simulink library "TriphaseHardwaremodule"  (R2019b)
settings: Solver=ode45  StartTime=0.0  StopTime=10.0  RelTol=1e-3
values from neighbouring files (symbols this model uses):
  ControlSampleTime = 1/8000    (= 0.000125)    [initTPHardware.m]
  HWSampleTime = ControlSampleTime / Oversample    [Sim_TP3_VSM_init.m]    (also in initTPHardware.m = 3.125e-05)
  L1 = 0    [initVirtualCircuit.m]
undefined symbols (not defined in the file or in its folder): C1, C2, C_cap, C_CM, C_damp, C_DC, DT, gcbh, Iac_bit, Iac_max, L2, L_CM, LCL, PWM_f, R_C1, R_C2, R_cap, R_damp, R_L1, R_L2, sps_rtmsupport, Vac_bit, Vac_max, Vdc_bit, Vdc_max
libraries: $bdroot x58, powerlib x46, triphase_hpc x7, powerlib_meascontrol x5, simulink x2
(part 1 of 3)
settings Model: Creator=fwelck  LastModifiedBy=e2n016
settings DataIOCC: LimitDataPoints=on  SaveFormat=Array  ReturnWorkspaceOutputs=off
settings OptimizationCC: BlockReduction=off  BooleanDataType=off  LifeSpan=inf
settings DebuggingCC: SaveWithParameterizedLinksMsg=none  UnderspecifiedInitializationDetection=Classic  MergeDetectMultiDrivingBlocksExec=none  SignalResolutionControl=TryResolveAllWithWarning  AllowSymbolicDim=off  SFUnexpectedBacktrackingDiag=warning  SFNoUnconditionalDefaultTransitionDiag=warning  SFExecutionAtInitializationDiag=none  ArithmeticOperatorsInVariantConditions=warning
settings HardwareCC: ProdBitPerPointer=32  ProdBitPerSizeT=32  ProdBitPerPtrDiffT=32  ProdLargestAtomicFloat=None  ProdIntDivRoundTo=Undefined  ProdEndianess=Unspecified  ProdWordSize=32  ProdHWDeviceType=32-bit Generic  TargetUnknown=on
settings ModelReferenceCC: PropagateSignalLabelsOutOfModel=off
settings SFSimCC: SimUseLocalCustomCode=off  CustomCodeUndefinedFunction=UseInterfaceOnly
settings RTWCC: RTWUseLocalCustomCode=off
settings CodeAppCC: StateflowObjectComments=on
settings GRTTargetCC: TargetLangStandard=C89/C90 (ANSI)  GeneratePreprocessorConditionals=Disable all
settings ConfigComp: CovMetricSettings=dw  CovHtmlReporting=on  CovSaveCumulativeToWorkspaceVar=on  CovSaveSingleToWorkspaceVar=on  CovExternalEMLEnable=off  CovSFcnEnable=off

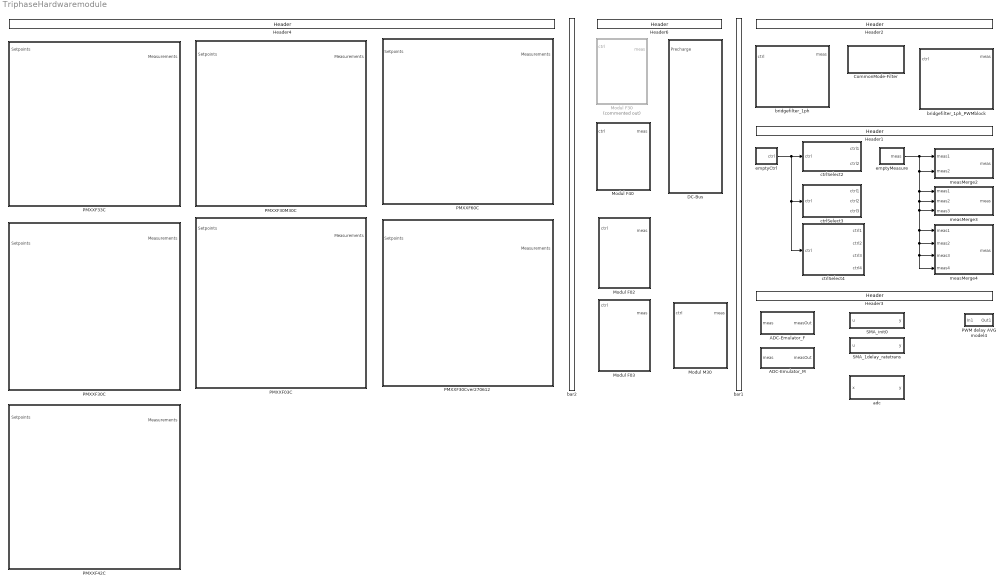
== system TriphaseHardwaremodule ==
  ADC-Emulator_F : Subsystem  mask{ADC_Emulation=off, ControlSampleTime=ControlSampleTime, HWSampleTime=HWSampleTime, Vac_max=Vac_max, Vac_bit=Vac_bit, Iac_max=Iac_max, Iac_bit=Iac_bit, Vdc_max=Vdc_max, Vdc_bit=Vdc_bit}
      mask prompts: Vac_max "AC Voltage Range"; Vac_bit "ADC resolution [bit]"; Iac_max "AC Current Range"; Iac_bit "ADC resolution [bit]"; Vdc_max "DC Voltage Range"; Vdc_bit "ADC resolution [bit]"
      mask init:
      | ParamValue=get_param(gcb,'ADC_Emulation');
      | set_param([gcb '/adc_i_inverter'],'ADC_Emulation',ParamValue);
      | set_param([gcb '/adc_i_out'],'ADC_Emulation',ParamValue);
      | set_param([gcb '/adc_u_cap'],'ADC_Emulation',ParamValue);
      | set_param([gcb '/adc_u_dc'],'ADC_Emulation',ParamValue);
      | set_param([gcb '/adc_u_out'],'ADC_Emulation',ParamValue);
      mask TypeOptions ADC_Emulation: off | on
      mask DialogControl GrpADC Prompt: ADC-Emulation
      mask DialogControl ADC_Text Prompt: ADC-emulation emulates the quantization resulting from AD-conversion. Moving Average is always applied over one ControlSampleTime
  ADC-Emulator_M : Subsystem  mask{ADC_Emulation=off, ControlSampleTime=ControlSampleTime, HWSampleTime=HWSampleTime, Vac_max=Vac_max, Vac_bit=Vac_bit, Iac_max=Iac_max, Iac_bit=Iac_bit, Vdc_max=Vdc_max, Vdc_bit=Vdc_bit}
      mask prompts: Vac_max "AC Voltage Range"; Vac_bit "ADC resolution [bit]"; Iac_max "AC Current Range"; Iac_bit "ADC resolution [bit]"; Vdc_max "DC Voltage Range"; Vdc_bit "ADC resolution [bit]"
      mask init:
      | ParamValue=get_param(gcb,'ADC_Emulation');
      | set_param([gcb '/adc_i_inverter'],'ADC_Emulation',ParamValue);
      | set_param([gcb '/adc_u_dc'],'ADC_Emulation',ParamValue);
      mask TypeOptions ADC_Emulation: off | on
      mask DialogControl GrpADC Prompt: ADC-Emulation
      mask DialogControl ADC_Text Prompt: ADC-emulation emulates the quantization resulting from AD-conversion. Moving Average is always applied over one ControlSampleTime
  CommonMode-Filter : Subsystem  mask{L_CM=L_CM, C_CM=C_CM, R_damp=R_damp, C_damp=C_damp}
      mask prompts: L_CM "Inductance [H]"; C_CM "Capacitance [F]"; R_damp "Damping resistance [Ohm]"; C_damp "Damping capacitance [F]"
      mask DialogControl GrpCM Prompt: Common-Mode
  DC-Bus : Subsystem  mask{C_cap=C_cap, R_cap=R_cap}
      mask prompts: C_cap "Capacitance [F]"; R_cap "Parallel Resistance [Ohm]"
      mask DialogControl GrpDC Prompt: DC-Bus
  Header1 : triphase_hpc/Utilities/Header  strCap=Signal Split and Merge  strColor=Dark Gray  strPen=white
  Header2 : triphase_hpc/Utilities/Header  strCap=Basic Inverter Modules  strColor=Dark Gray  strPen=white
  Header3 : triphase_hpc/Utilities/Header  strCap=ADC Modules  strColor=Dark Gray  strPen=white
  Header4 : triphase_hpc/Utilities/Header  strCap=Triphase Hardware  strColor=Dark Gray  strPen=white
  Header6 : triphase_hpc/Utilities/Header  strCap=Basic Triphase Modules  strColor=Dark Gray  strPen=white
  Modul F02 : Subsystem  mask{Leistungsklasse=Custom, LCFilterChoice=LC, L1=L1, R_L1=R_L1, C1=C1, R_C1=R_C1, L2=L2, R_L2=R_L2, C2=C2, R_C2=R_C2, PWM_f=PWM_f, DT=DT, ADC_Emulation=off, ControlSampleTime=ControlSampleTime, HWSampleTime=HWSampleTime, Vac_max=Vac_max, Vac_bit=Vac_bit, Iac_max=Iac_max, Iac_bit=Iac_bit, Vdc_max=Vdc_max, Vdc_bit=Vdc_bit}
      mask prompts: LCFilterChoice "AC-Filter"; L1 "Inductance L1 [H]"; R_L1 "Series resistance of L1 [Ohm]"; C1 "Capacitance C1 [F]"; R_C1 "Series resistance of C1 [Ohm]"; L2 "Inductance L2 [H]"; R_L2 "Series resistance of L2 [Ohm]"; C2 "Capacitance C2 [F]"; R_C2 "Series resistance of C2 [Ohm]"; PWM_f "PWM Frequency"; DT "On Delay"; Vac_max "AC Voltage Range"; Vac_bit "ADC resolution [bit]"; Iac_max "AC Current Range"; Iac_bit "ADC resolution [bit]"; Vdc_max "DC Voltage Range"; Vdc_bit "ADC resolution [bit]"
      mask init:
      | ParamValue=get_param(gcb,'ADC_Emulation');
      | set_param([gcb '/ADC-Emulator_F'],'ADC_Emulation',ParamValue);
      | 
      | ParamValue=get_param(gcb,'LCFilterChoice');
      | set_param([gcb '/bridgefilter_dca'],'LCFilterChoice',ParamValue);
      | set_param([gcb '/bridgefilter_dcb'],'LCFilterChoice',ParamValue);
      mask TypeOptions Leistungsklasse: 5kW | 15kW | 90kW | Custom
      mask Callback Leistungsklasse: loadTriphaseHardwareParameter
      mask TypeOptions LCFilterChoice: LC | LCL | LCC | LCLC
      mask TypeOptions ADC_Emulation: off | on
      mask DialogControl GrpLoad Prompt: Triphase
      mask DialogControl LC Prompt: LC(L)(C)
      mask DialogControl GrpLC Prompt: LC(L)(C)-Filter
      mask DialogControl SW Prompt: Swichted
      mask DialogControl GrpSW Prompt: Switched
      mask DialogControl ADC Prompt: ADC
      mask DialogControl GrpADC Prompt: ADC-Emulation
      mask DialogControl ADC_Text Prompt: ADC-emulation emulates the quantization resulting from AD-conversion. Moving Average is always applied over one ControlSampleTime
  Modul F03 : Subsystem  mask{Leistungsklasse=Custom, LCFilterChoice=LC, L1=L1, R_L1=R_L1, C1=C1, R_C1=R_C1, L2=L2, R_L2=R_L2, C2=C2, R_C2=R_C2, PWM_f=PWM_f, DT=DT, ADC_Emulation=off, ControlSampleTime=ControlSampleTime, HWSampleTime=HWSampleTime, Vac_max=Vac_max, Vac_bit=Vac_bit, Iac_max=Iac_max, Iac_bit=Iac_bit, Vdc_max=Vdc_max, Vdc_bit=Vdc_bit}
      mask prompts: LCFilterChoice "AC-Filter"; L1 "Inductance L1 [H]"; R_L1 "Series resistance of L1 [Ohm]"; C1 "Capacitance C1 [F]"; R_C1 "Series resistance of C1 [Ohm]"; L2 "Inductance L2 [H]"; R_L2 "Series resistance of L2 [Ohm]"; C2 "Capacitance C2 [F]"; R_C2 "Series resistance of C2 [Ohm]"; PWM_f "PWM Frequency"; DT "On Delay"; Vac_max "AC Voltage Range"; Vac_bit "ADC resolution [bit]"; Iac_max "AC Current Range"; Iac_bit "ADC resolution [bit]"; Vdc_max "DC Voltage Range"; Vdc_bit "ADC resolution [bit]"
      mask init:
      | ParamValue=get_param(gcb,'ADC_Emulation');
      | set_param([gcb '/ADC-Emulator_F'],'ADC_Emulation',ParamValue);
      | 
      | ParamValue=get_param(gcb,'LCFilterChoice');
      | set_param([gcb '/bridgefilter_dca'],'LCFilterChoice',ParamValue);
      | set_param([gcb '/bridgefilter_dcb'],'LCFilterChoice',ParamValue);
      | set_param([gcb '/bridgefilter_dcb1'],'LCFilterChoice',ParamValue);
      mask TypeOptions Leistungsklasse: 5kW | 15kW | 90kW | Custom
      mask Callback Leistungsklasse: loadTriphaseHardwareParameter
      mask TypeOptions LCFilterChoice: LC | LCL | LCC | LCLC
      mask TypeOptions ADC_Emulation: off | on
      mask DialogControl GrpLoad Prompt: Triphase
      mask DialogControl LC Prompt: LC(L)(C)
      mask DialogControl GrpLC Prompt: LC(L)(C)-Filter
      mask DialogControl SW Prompt: Swichted
      mask DialogControl GrpSW Prompt: Switched
      mask DialogControl ADC Prompt: ADC
      mask DialogControl GrpADC Prompt: ADC-Emulation
      mask DialogControl ADC_Text Prompt: ADC-emulation emulates the quantization resulting from AD-conversion. Moving Average is always applied over one ControlSampleTime
  Modul F30 : Subsystem  Commented=on  mask{Leistungsklasse=Custom, LCFilterChoice=LCLC, L1=L1, R_L1=R_L1, C1=C1, R_C1=R_C1, L2=L2, R_L2=R_L2, C2=C2, R_C2=R_C2, PWM_f=PWM_f, DT=DT, ADC_Emulation=off, ControlSampleTime=ControlSampleTime, HWSampleTime=HWSampleTime, Vac_max=Vac_max, Vac_bit=Vac_bit, Iac_max=Iac_max, Iac_bit=Iac_bit, Vdc_max=Vdc_max, Vdc_bit=Vdc_bit}
      mask prompts: LCFilterChoice "AC-Filter"; L1 "Inductance L1 [H]"; R_L1 "Series resistance of L1 [Ohm]"; C1 "Capacitance C1 [F]"; R_C1 "Series resistance of C1 [Ohm]"; L2 "Inductance L2 [H]"; R_L2 "Series resistance of L2 [Ohm]"; C2 "Capacitance C2 [F]"; R_C2 "Series resistance of C2 [Ohm]"; PWM_f "PWM Frequency"; DT "On Delay"; Vac_max "AC Voltage Range"; Vac_bit "ADC resolution [bit]"; Iac_max "AC Current Range"; Iac_bit "ADC resolution [bit]"; Vdc_max "DC Voltage Range"; Vdc_bit "ADC resolution [bit]"
      mask init:
      | ParamValue=get_param(gcb,'ADC_Emulation');
      | set_param([gcb '/ADC-Emulator_F'],'ADC_Emulation',ParamValue);
      | 
      | ParamValue=get_param(gcb,'LCFilterChoice');
      | set_param([gcb '/bridgefilter_aca'],'LCFilterChoice',ParamValue);
      | set_param([gcb '/bridgefilter_acb'],'LCFilterChoice',ParamValue);
      | set_param([gcb '/bridgefilter_acc'],'LCFilterChoice',ParamValue);
      mask TypeOptions Leistungsklasse: 5kW | 15kW | 90kW | Custom
      mask Callback Leistungsklasse: loadTriphaseHardwareParameter
      mask TypeOptions LCFilterChoice: LC | LCL | LCC | LCLC
      mask TypeOptions ADC_Emulation: off | on
      mask DialogControl GrpLoad Prompt: Triphase
      mask DialogControl LC Prompt: LC(L)(C)
      mask DialogControl GrpLC Prompt: LC(L)(C)-Filter
      mask DialogControl SW Prompt: Swichted
      mask DialogControl GrpSW Prompt: Switched
      mask DialogControl ADC Prompt: ADC
      mask DialogControl GrpADC Prompt: ADC-Emulation
      mask DialogControl ADC_Text Prompt: ADC-emulation emulates the quantization resulting from AD-conversion. Moving Average is always applied over one ControlSampleTime
  Modul F40 : Subsystem  mask{Leistungsklasse=Custom, LCFilterChoice=LC, L1=L1, R_L1=R_L1, C1=C1, R_C1=R_C1, L2=L2, R_L2=R_L2, C2=C2, R_C2=R_C2, PWM_f=PWM_f, DT=DT, ADC_Emulation=off, ControlSampleTime=ControlSampleTime, HWSampleTime=HWSampleTime, Vac_max=Vac_max, Vac_bit=Vac_bit, Iac_max=Iac_max, Iac_bit=Iac_bit, Vdc_max=Vdc_max, Vdc_bit=Vdc_bit}
      mask prompts: LCFilterChoice "AC-Filter"; L1 "Inductance L1 [H]"; R_L1 "Series resistance of L1 [Ohm]"; C1 "Capacitance C1 [F]"; R_C1 "Series resistance of C1 [Ohm]"; L2 "Inductance L2 [H]"; R_L2 "Series resistance of L2 [Ohm]"; C2 "Capacitance C2 [F]"; R_C2 "Series resistance of C2 [Ohm]"; PWM_f "PWM Frequency"; DT "On Delay"; Vac_max "AC Voltage Range"; Vac_bit "ADC resolution [bit]"; Iac_max "AC Current Range"; Iac_bit "ADC resolution [bit]"; Vdc_max "DC Voltage Range"; Vdc_bit "ADC resolution [bit]"
      mask init:
      | ParamValue=get_param(gcb,'ADC_Emulation');
      | set_param([gcb '/ADC-Emulator_F'],'ADC_Emulation',ParamValue);
      | 
      | ParamValue=get_param(gcb,'LCFilterChoice');
      | set_param([gcb '/bridgefilter_aca'],'LCFilterChoice',ParamValue);
      | set_param([gcb '/bridgefilter_acb'],'LCFilterChoice',ParamValue);
      | set_param([gcb '/bridgefilter_acc'],'LCFilterChoice',ParamValue);
      | set_param([gcb '/bridgefilter_acd'],'LCFilterChoice',ParamValue);
      mask TypeOptions Leistungsklasse: 5kW | 15kW | 90kW | Custom
      mask Callback Leistungsklasse: loadTriphaseHardwareParameter
      mask TypeOptions LCFilterChoice: LC | LCL | LCC | LCLC
      mask TypeOptions ADC_Emulation: off | on
      mask DialogControl GrpLoad Prompt: Triphase
      mask DialogControl LC Prompt: LC(L)(C)
      mask DialogControl GrpLC Prompt: LC(L)(C)-Filter
      mask DialogControl SW Prompt: Swichted
      mask DialogControl GrpSW Prompt: Switched
      mask DialogControl ADC Prompt: ADC
      mask DialogControl GrpADC Prompt: ADC-Emulation
      mask DialogControl ADC_Text Prompt: ADC-emulation emulates the quantization resulting from AD-conversion. Moving Average is always applied over one ControlSampleTime
  Modul M30 : Subsystem  mask{PWM_f=PWM_f, DT=DT}
      mask prompts: PWM_f "PWM Frequency"; DT "On Delay"
      mask DialogControl GrpSW Prompt: Switched
  PMXXF03C : Subsystem  VariantControl=PMXXF03C  mask{Leistungsklasse=Custom, LCFilterChoice=LC, L1=L1, R_L1=R_L1, C1=C1, R_C1=R_C1, L2=L2, R_L2=R_L2, C2=C2, R_C2=R_C2, C_cap=C_cap, R_cap=R_cap, PWM_f=PWM_f, DT=DT, ADC_Emulation=off, ControlSampleTime=ControlSampleTime, HWSampleTime=HWSampleTime, Vac_max=Vac_max, Vac_bit=Vac_bit, Iac_max=Iac_max, Iac_bit=Iac_bit, Vdc_max=Vdc_max, Vdc_bit=Vdc_bit}
      mask prompts: LCFilterChoice "AC-Filter"; L1 "Inductance L1 [H]"; R_L1 "Series resistance of L1 [Ohm]"; C1 "Capacitance C1 [F]"; R_C1 "Series resistance of C1 [Ohm]"; L2 "Inductance L2 [H]"; R_L2 "Series resistance of L2 [Ohm]"; C2 "Capacitance C2 [F]"; R_C2 "Series resistance of C2 [Ohm]"; C_cap "Capacitance [F]"; R_cap "Parallel Resistance [Ohm]"; PWM_f "PWM Frequency"; DT "On Delay"; Vac_max "AC Voltage Range"; Vac_bit "ADC resolution [bit]"; Iac_max "AC Current Range"; Iac_bit "ADC resolution [bit]"; Vdc_max "DC Voltage Range"; Vdc_bit "ADC resolution [bit]"
      mask init:
      | ParamValue=get_param(gcb,'ADC_Emulation');
      | set_param([gcb '/Modul F03'],'ADC_Emulation',ParamValue);
      | 
      | ParamValue=get_param(gcb,'LCFilterChoice');
      | set_param([gcb '/Modul F03'],'LCFilterChoice',ParamValue);
      mask TypeOptions Leistungsklasse: 5kW | 15kW | 90kW | Custom
      mask Callback Leistungsklasse: loadTriphaseHardwareParameter
      mask TypeOptions LCFilterChoice: LC | LCL | LCC | LCLC
      mask TypeOptions ADC_Emulation: off | on
      mask DialogControl GrpLoad Prompt: Triphase
      mask DialogControl HW1 Prompt: Hardware (1)
      mask DialogControl GrpLC Prompt: LC(L)(C)-Filter
      mask DialogControl HW2 Prompt: Hardware (2)
      mask DialogControl GrpDC Prompt: DC-Bus
      mask DialogControl GrpSW Prompt: Switched
      mask DialogControl HW3 Prompt: Hardware (3)
      mask DialogControl GrpADC Prompt: ADC-Emulation
      mask DialogControl ADC_Text Prompt: ADC-emulation emulates the quantization resulting from AD-conversion. Moving Average is always applied over one ControlSampleTime
  PMXXF30C : Subsystem  VariantControl=PMXXF30C  mask{Leistungsklasse=Custom, LCFilterChoice=LC, L1=L1, R_L1=R_L1, C1=C1, R_C1=R_C1, L2=L2, R_L2=R_L2, C2=C2, R_C2=R_C2, C_cap=C_cap, R_cap=R_cap, PWM_f=PWM_f, DT=DT, ADC_Emulation=off, ControlSampleTime=ControlSampleTime, HWSampleTime=HWSampleTime, Vac_max=Vac_max, Vac_bit=Vac_bit, Iac_max=Iac_max, Iac_bit=Iac_bit, Vdc_max=Vdc_max, Vdc_bit=Vdc_bit}
      mask prompts: LCFilterChoice "AC-Filter"; L1 "Inductance L1 [H]"; R_L1 "Series resistance of L1 [Ohm]"; C1 "Capacitance C1 [F]"; R_C1 "Series resistance of C1 [Ohm]"; L2 "Inductance L2 [H]"; R_L2 "Series resistance of L2 [Ohm]"; C2 "Capacitance C2 [F]"; R_C2 "Series resistance of C2 [Ohm]"; C_cap "Capacitance [F]"; R_cap "Parallel Resistance [Ohm]"; PWM_f "PWM Frequency"; DT "On Delay"; Vac_max "AC Voltage Range"; Vac_bit "ADC resolution [bit]"; Iac_max "AC Current Range"; Iac_bit "ADC resolution [bit]"; Vdc_max "DC Voltage Range"; Vdc_bit "ADC resolution [bit]"
      mask init:
      | ParamValue=get_param(gcb,'ADC_Emulation');
      | set_param([gcb '/Modul F30'],'ADC_Emulation',ParamValue);
      | 
      | ParamValue=get_param(gcb,'LCFilterChoice');
      | set_param([gcb '/Modul F30'],'LCFilterChoice',ParamValue);
      mask TypeOptions Leistungsklasse: 5kW | 15kW | 90kW | Custom
      mask Callback Leistungsklasse: loadTriphaseHardwareParameter
      mask TypeOptions LCFilterChoice: LC | LCL | LCC | LCLC
      mask TypeOptions ADC_Emulation: off | on
      mask DialogControl GrpLoad Prompt: Triphase
      mask DialogControl HW1 Prompt: Hardware (1)
      mask DialogControl GrpLC Prompt: LC(L)(C)-Filter
      mask DialogControl HW2 Prompt: Hardware (2)
      mask DialogControl GrpDC Prompt: DC-Bus
      mask DialogControl GrpSW Prompt: Switched
      mask DialogControl HW3 Prompt: Hardware (3)
      mask DialogControl GrpADC Prompt: ADC-Emulation
      mask DialogControl ADC_Text Prompt: ADC-emulation emulates the quantization resulting from AD-conversion. Moving Average is always applied over one ControlSampleTime
  PMXXF30Cver270612 : Subsystem  VariantControl=PMXXF30Cver270612  mask{Leistungsklasse=Custom, LCFilterChoice=LC, L1=L1, R_L1=R_L1, C1=C1, R_C1=R_C1, L2=L2, R_L2=R_L2, C2=C2, R_C2=R_C2, C_cap=C_cap, R_cap=R_cap, PWM_f=PWM_f, DT=DT, ADC_Emulation=off, ControlSampleTime=ControlSampleTime, HWSampleTime=HWSampleTime, Vac_max=Vac_max, Vac_bit=Vac_bit, Iac_max=Iac_max, Iac_bit=Iac_bit, Vdc_max=Vdc_max, Vdc_bit=Vdc_bit}
      mask prompts: LCFilterChoice "AC-Filter"; L1 "Inductance L1 [H]"; R_L1 "Series resistance of L1 [Ohm]"; C1 "Capacitance C1 [F]"; R_C1 "Series resistance of C1 [Ohm]"; L2 "Inductance L2 [H]"; R_L2 "Series resistance of L2 [Ohm]"; C2 "Capacitance C2 [F]"; R_C2 "Series resistance of C2 [Ohm]"; C_cap "Capacitance [F]"; R_cap "Parallel Resistance [Ohm]"; PWM_f "PWM Frequency"; DT "On Delay"; Vac_max "AC Voltage Range"; Vac_bit "ADC resolution [bit]"; Iac_max "AC Current Range"; Iac_bit "ADC resolution [bit]"; Vdc_max "DC Voltage Range"; Vdc_bit "ADC resolution [bit]"
      mask init: same as TriphaseHardwaremodule/PMXXF30C
      mask TypeOptions Leistungsklasse: 5kW | 15kW | 90kW | Custom
      mask Callback Leistungsklasse: loadTriphaseHardwareParameter
      mask TypeOptions LCFilterChoice: LC | LCL | LCC | LCLC
      mask TypeOptions ADC_Emulation: off | on
      mask DialogControl GrpLoad Prompt: Triphase
      mask DialogControl HW1 Prompt: Hardware (1)
      mask DialogControl GrpLC Prompt: LC(L)(C)-Filter
      mask DialogControl HW2 Prompt: Hardware (2)
      mask DialogControl GrpDC Prompt: DC-Bus
      mask DialogControl GrpSW Prompt: Switched
      mask DialogControl HW3 Prompt: Hardware (3)
      mask DialogControl GrpADC Prompt: ADC-Emulation
      mask DialogControl ADC_Text Prompt: ADC-emulation emulates the quantization resulting from AD-conversion. Moving Average is always applied over one ControlSampleTime
  PMXXF30M30C : Subsystem  VariantControl=PMXXF30M30C  mask{Leistungsklasse=Custom, LCFilterChoice=LC, L1=L1, R_L1=R_L1, C1=C1, R_C1=R_C1, L2=L2, R_L2=R_L2, C2=C2, R_C2=R_C2, C_cap=C_cap, R_cap=R_cap, PWM_f=PWM_f, DT=DT, ADC_Emulation=off, ControlSampleTime=ControlSampleTime, HWSampleTime=HWSampleTime, Vac_max=Vac_max, Vac_bit=Vac_bit, Iac_max=Iac_max, Iac_bit=Iac_bit, Vdc_max=Vdc_max, Vdc_bit=Vdc_bit}
      mask prompts: LCFilterChoice "AC-Filter"; L1 "Inductance L1 [H]"; R_L1 "Series resistance of L1 [Ohm]"; C1 "Capacitance C1 [F]"; R_C1 "Series resistance of C1 [Ohm]"; L2 "Inductance L2 [H]"; R_L2 "Series resistance of L2 [Ohm]"; C2 "Capacitance C2 [F]"; R_C2 "Series resistance of C2 [Ohm]"; C_cap "Capacitance [F]"; R_cap "Parallel Resistance [Ohm]"; PWM_f "PWM Frequency"; DT "On Delay"; Vac_max "AC Voltage Range"; Vac_bit "ADC resolution [bit]"; Iac_max "AC Current Range"; Iac_bit "ADC resolution [bit]"; Vdc_max "DC Voltage Range"; Vdc_bit "ADC resolution [bit]"
      mask init: same as TriphaseHardwaremodule/PMXXF30C
      mask TypeOptions Leistungsklasse: 5kW | 15kW | 90kW | Custom
      mask Callback Leistungsklasse: loadTriphaseHardwareParameter
      mask TypeOptions LCFilterChoice: LC | LCL | LCC | LCLC
      mask TypeOptions ADC_Emulation: off | on
      mask DialogControl GrpLoad Prompt: Triphase
      mask DialogControl HW1 Prompt: Hardware (1)
      mask DialogControl GrpLC Prompt: LC(L)(C)-Filter
      mask DialogControl HW2 Prompt: Hardware (2)
      mask DialogControl GrpDC Prompt: DC-Bus
      mask DialogControl GrpSW Prompt: Switched
      mask DialogControl HW3 Prompt: Hardware (3)
      mask DialogControl GrpADC Prompt: ADC-Emulation
      mask DialogControl ADC_Text Prompt: ADC-emulation emulates the quantization resulting from AD-conversion. Moving Average is always applied over one ControlSampleTime
  PMXXF33C : Subsystem  VariantControl=PMXXF33C  mask{Leistungsklasse=Custom, LCFilterChoice1=LCLC, LCFilterChoice2=LC, L1=LCL.SI.L1, R_L1=LCL.SI.R1, C1=LCL.SI.C, R_C1=LCL.SI.Rc, L2=LCL.SI.L2, R_L2=LCL.SI.R2, C2=LCL.SI.C/10, R_C2=LCL.SI.Rc, C_cap=2e-3%720e-6/2, R_cap=1000000, PWM_f=1/ControlSampleTime, DT=300e-09, ADC_Emulation=off, ControlSampleTime=ControlSampleTime, HWSampleTime=HWSampleTime, Vac_max=1000, Vac_bit=16, Iac_max=400, Iac_bit=16, Vdc_max=1000, Vdc_bit=16}
      mask prompts: LCFilterChoice1 "AC-Filter 1"; LCFilterChoice2 "AC-Filter 2"; L1 "Inductance L1 [H]"; R_L1 "Series resistance of L1 [Ohm]"; C1 "Capacitance C1 [F]"; R_C1 "Series resistance of C1 [Ohm]"; L2 "Inductance L2 [H]"; R_L2 "Series resistance of L2 [Ohm]"; C2 "Capacitance C2 [F]"; R_C2 "Series resistance of C2 [Ohm]"; C_cap "Capacitance [F]"; R_cap "Parallel Resistance [Ohm]"; PWM_f "PWM Frequency"; DT "On Delay"; Vac_max "AC Voltage Range"; Vac_bit "ADC resolution [bit]"; Iac_max "AC Current Range"; Iac_bit "ADC resolution [bit]"; Vdc_max "DC Voltage Range"; Vdc_bit "ADC resolution [bit]"
      mask init:
      | ParamValue=get_param(gcb,'ADC_Emulation');
      | set_param([gcb '/Modul F30'],'ADC_Emulation',ParamValue);
      | set_param([gcb '/Modul F03'],'ADC_Emulation',ParamValue);
      | 
      | ParamValue=get_param(gcb,'LCFilterChoice1');
      | set_param([gcb '/Modul F30'],'LCFilterChoice',ParamValue);
      | ParamValue=get_param(gcb,'LCFilterChoice2');
      | set_param([gcb '/Modul F03'],'LCFilterChoice',ParamValue);
      mask TypeOptions Leistungsklasse: 5kW | 15kW | 90kW | Custom
      mask Callback Leistungsklasse: loadTriphaseHardwareParameter
      mask TypeOptions LCFilterChoice1: LC | LCL | LCC | LCLC
      mask TypeOptions LCFilterChoice2: LC | LCL | LCC | LCLC
      mask TypeOptions ADC_Emulation: off | on
      mask DialogControl GrpLoad Prompt: Triphase
      mask DialogControl HW1 Prompt: Hardware (1)
      mask DialogControl GrpLC Prompt: LC(L)(C)-Filter
      mask DialogControl HW2 Prompt: Hardware (2)
      mask DialogControl GrpDC Prompt: DC-Bus
      mask DialogControl GrpSW Prompt: Switched
      mask DialogControl HW3 Prompt: Hardware (3)
      mask DialogControl GrpADC Prompt: ADC-Emulation
      mask DialogControl ADC_Text Prompt: ADC-emulation emulates the quantization resulting from AD-conversion. Moving Average is always applied over one ControlSampleTime
  PMXXF42C : Subsystem  VariantControl=PMXXF33C  mask{Leistungsklasse=Custom, LCFilterChoice1=LC, LCFilterChoice2=LC, L1=L1, R_L1=R_L1, C1=C1, R_C1=R_C1, L2=L2, R_L2=R_L2, C2=C2, R_C2=R_C2, C_cap=C_cap, R_cap=R_cap, PWM_f=PWM_f, DT=DT, ADC_Emulation=off, ControlSampleTime=ControlSampleTime, HWSampleTime=HWSampleTime, Vac_max=Vac_max, Vac_bit=Vac_bit, Iac_max=Iac_max, Iac_bit=Iac_bit, Vdc_max=Vdc_max, Vdc_bit=Vdc_bit}
      mask prompts: LCFilterChoice1 "AC-Filter 1"; LCFilterChoice2 "AC-Filter 2"; L1 "Inductance L1 [H]"; R_L1 "Series resistance of L1 [Ohm]"; C1 "Capacitance C1 [F]"; R_C1 "Series resistance of C1 [Ohm]"; L2 "Inductance L2 [H]"; R_L2 "Series resistance of L2 [Ohm]"; C2 "Capacitance C2 [F]"; R_C2 "Series resistance of C2 [Ohm]"; C_cap "Capacitance [F]"; R_cap "Parallel Resistance [Ohm]"; PWM_f "PWM Frequency"; DT "On Delay"; Vac_max "AC Voltage Range"; Vac_bit "ADC resolution [bit]"; Iac_max "AC Current Range"; Iac_bit "ADC resolution [bit]"; Vdc_max "DC Voltage Range"; Vdc_bit "ADC resolution [bit]"
      mask init:
      | ParamValue=get_param(gcb,'ADC_Emulation');
      | set_param([gcb '/Modul F02'],'ADC_Emulation',ParamValue);
      | set_param([gcb '/Modul F40'],'ADC_Emulation',ParamValue);
      | 
      | ParamValue1=get_param(gcb,'LCFilterChoice1');
      | ParamValue2=get_param(gcb,'LCFilterChoice2');
      | set_param([gcb '/Modul F40'],'LCFilterChoice',ParamValue1);
      | set_param([gcb '/Modul F02'],'LCFilterChoice',ParamValue2);
      mask TypeOptions Leistungsklasse: 5kW | 15kW | 90kW | Custom
      mask Callback Leistungsklasse: loadTriphaseHardwareParameter
      mask TypeOptions LCFilterChoice1: LC | LCL | LCC | LCLC
      mask TypeOptions LCFilterChoice2: LC | LCL | LCC | LCLC
      mask TypeOptions ADC_Emulation: off | on
      mask DialogControl GrpLoad Prompt: Triphase
      mask DialogControl HW1 Prompt: Hardware (1)
      mask DialogControl GrpLC Prompt: LC(L)(C)-Filter
      mask DialogControl HW2 Prompt: Hardware (2)
      mask DialogControl GrpDC Prompt: DC-Bus
      mask DialogControl GrpSW Prompt: Switched
      mask DialogControl HW3 Prompt: Hardware (3)
      mask DialogControl GrpADC Prompt: ADC-Emulation
      mask DialogControl ADC_Text Prompt: ADC-emulation emulates the quantization resulting from AD-conversion. Moving Average is always applied over one ControlSampleTime
  PMXXF60C : Subsystem  VariantControl=PMXXF60C  mask{Leistungsklasse=Custom, LCFilterChoice1=LC, LCFilterChoice2=LC, L1=LCL.SI.L1, R_L1=LCL.SI.R1, C1=LCL.SI.C, R_C1=LCL.SI.Rc, L2=LCL.SI.L2, R_L2=LCL.SI.R2, C2=LCL.SI.C, R_C2=LCL.SI.Rc, C_cap=0.0018, R_cap=1000000, PWM_f=8000, DT=1e-06, ADC_Emulation=off, ControlSampleTime=ControlSampleTime, HWSampleTime=HWSampleTime, Vac_max=1000, Vac_bit=16, Iac_max=400, Iac_bit=16, Vdc_max=1000, Vdc_bit=16}
      mask prompts: LCFilterChoice1 "AC-Filter 1"; LCFilterChoice2 "AC-Filter 2"; L1 "Inductance L1 [H]"; R_L1 "Series resistance of L1 [Ohm]"; C1 "Capacitance C1 [F]"; R_C1 "Series resistance of C1 [Ohm]"; L2 "Inductance L2 [H]"; R_L2 "Series resistance of L2 [Ohm]"; C2 "Capacitance C2 [F]"; R_C2 "Series resistance of C2 [Ohm]"; C_cap "Capacitance [F]"; R_cap "Parallel Resistance [Ohm]"; PWM_f "PWM Frequency"; DT "On Delay"; Vac_max "AC Voltage Range"; Vac_bit "ADC resolution [bit]"; Iac_max "AC Current Range"; Iac_bit "ADC resolution [bit]"; Vdc_max "DC Voltage Range"; Vdc_bit "ADC resolution [bit]"
      mask init:
      | ParamValue=get_param(gcb,'ADC_Emulation');
      | set_param([gcb '/Modul F30_1'],'ADC_Emulation',ParamValue);
      | set_param([gcb '/Modul F30_2'],'ADC_Emulation',ParamValue);
      | 
      | ParamValue1=get_param(gcb,'LCFilterChoice1');
      | ParamValue2=get_param(gcb,'LCFilterChoice2');
      | set_param([gcb '/Modul F30_1'],'LCFilterChoice',ParamValue1);
      | set_param([gcb '/Modul F30_2'],'LCFilterChoice',ParamValue2);
      mask TypeOptions Leistungsklasse: 5kW | 15kW | 90kW | Custom
      mask Callback Leistungsklasse: loadTriphaseHardwareParameter
      mask TypeOptions LCFilterChoice1: LC | LCL | LCC | LCLC
      mask TypeOptions LCFilterChoice2: LC | LCL | LCC | LCLC
      mask TypeOptions ADC_Emulation: off | on
      mask DialogControl GrpLoad Prompt: Triphase
      mask DialogControl HW1 Prompt: Hardware (1)
      mask DialogControl GrpLC Prompt: LC(L)(C)-Filter
      mask DialogControl HW2 Prompt: Hardware (2)
      mask DialogControl GrpDC Prompt: DC-Bus
      mask DialogControl GrpSW Prompt: Switched
      mask DialogControl HW3 Prompt: Hardware (3)
      mask DialogControl GrpADC Prompt: ADC-Emulation
      mask DialogControl ADC_Text Prompt: ADC-emulation emulates the quantization resulting from AD-conversion. Moving Average is always applied over one ControlSampleTime
  PWM delay AVG model4 : Subsystem
  SMA_1delay_ratetrans : Subsystem  mask{n_samples=round(ControlSampleTime/HWSampleTime), SlowSampleTime=ControlSampleTime}
      mask prompts: n_samples "Number of samples to average over"; SlowSampleTime "Output sample time"
      mask DialogControl DescGroupVar Prompt: Simple Moving Average
      mask DialogControl DescTextVar Prompt: Cycle buffer implementation of a simple moving average with initialization. Performs a lot faster than a FIR implementation for averages of 3 or more samples.
  SMA_init0 : Subsystem  mask{n_samples=round(ControlSampleTime/HWSampleTime)}
      mask prompts: n_samples "Number of samples to average over"
      mask DialogControl DescGroupVar Prompt: Simple Moving Average
      mask DialogControl DescTextVar Prompt: Cycle buffer implementation of a simple moving average with initialization. Performs a lot faster than a FIR implementation for averages of 3 or more samples.
  adc : Subsystem  mask(ADC Emulation){ADC_Emulation=off, ControlSampleTime=1, HWSampleTime=1, MeasMax=1, MeasBits=1}
      mask TypeOptions ADC_Emulation: off | on
      mask Display: fprintf(['ADC: ' get_param(gcb,'ADC_Emulation')])
  bar1 : triphase_hpc/Utilities/bar
  bar2 : triphase_hpc/Utilities/bar
  bridgefilter_1ph : Subsystem  mask{LCFilterChoice=LC, L1=L1, R_L1=R_L1, C1=C1, R_C1=R_C1, L2=L2, R_L2=R_L2, C2=C2, R_C2=R_C2, PWM_f=PWM_f, DT=DT}
      mask prompts: LCFilterChoice "AC-Filter"; L1 "Inductance L1 [H]"; R_L1 "Series resistance of L1 [Ohm]"; C1 "Capacitance C1 [F]"; R_C1 "Series resistance of C1 [Ohm]"; L2 "Inductance L2 [H]"; R_L2 "Series resistance of L2 [Ohm]"; C2 "Capacitance C2 [F]"; R_C2 "Series resistance of C2 [Ohm]"; PWM_f "PWM Frequency"; DT "On Delay"
      mask init:
      | switch get_param(gcb,'LCFilterChoice')
      |     case 'LC'
      |         LCFilterString='LC';
      |         IS_L2=false;
      |         IS_C2=false;
      |     case 'LCL'
      |         LCFilterString='LCL';
      |         IS_L2=true;
      |         IS_C2=false;
      |     case 'LCC'
      |         LCFilterString='LCC';
      |         IS_L2=false;
      |         IS_C2=true;
      |     case 'LCLC'
      |         LCFilterString='LCLC';
      |         IS_L2=true;
      |         IS_C2=true;
      | end
      | 
      | if IS_L2
      |     set_param([gcb '/L2'],'BranchType','RL','Resistance','R_L2')
      | else
      |     set_param([gcb '/L2'],'BranchType','R','Resistance','0.001')
      | end
      | 
      | if IS_C2
      |     set_param([gcb '/C2'],'BranchType','RC')
      | else
      |     set_param([gcb '/C2'],'BranchType','Open circuit')
      | end
      mask TypeOptions LCFilterChoice: LC | LCL | LCC | LCLC
      mask DialogControl LC Prompt: LC(L)(C)
      mask DialogControl GrpLC Prompt: LC(L)(C)-Filter
      mask DialogControl SW Prompt: Swichted
      mask DialogControl GrpSW Prompt: Switched
      mask Display:
      | IS_L1=true;
      | IS_C1=true;
      | switch get_param(gcb,'LCFilterChoice');
      |     case 'LC'
      |         LCFilterString='LC';
      |         IS_L2=false;
      |         IS_C2=false;
      |     case 'LCL'
      |         LCFilterString='LCL';
      |         IS_L2=true;
      |         IS_C2=false;
      |     case 'LCC'
      |         LCFilterString='LCC';
      |         IS_L2=false;
      |         IS_C2=true;
      |     case 'LCLC'
      |         LCFilterString='LCLC';
      |         IS_L2=true;
      |         IS_C2=true;
      |     otherwise
      |         LCFilterString='LC';
      |         IS_L2=false;
      |         IS_C2=false;
      | end
      | 
      | x0=10;
      | y0=25;
      | w=20;%Breite der Bauelemente
      | h=5;%Höhe der Bauelemente
      | 
      | x1 = linspace(0,1,50);
      | y1 = h*abs(sin(4*pi*x1));
      | 
      | plot(0,0);
      | plot(4*w+4*x0+50,150);
      | 
      | plot(0*w+x0+[0 x0],(100-y0)*[1 1]);
      | plot(0*w+2*x0+[0 w],(100-y0)*[1 1]);
      | if IS_L2
      |     plot(1*w+2*x0+w*x1, y1+100-y0);
      | else
      |     plot(1*w+2*x0+[0 w],(100-y0)*[1 1]);
      | end
      | plot(2*w+2*x0+[0 w],(100-y0)*[1 1]);
      | if IS_L1
      |     plot(3*w+2*x0+w*x1,y1+100-y0);
      | else
      |     plot(3*w+2*x0+[0 w],(100-y0)*[1 1]);
      | end
      | plot(4*w+2*x0+[0 x0],(100-y0)*[1 1]);
      | plot(x0+[0 x0],(y0)*[1 1]);
      | plot(w+x0+[0 7*w],(y0)*[1 1]);
      | 
      | %text(2*w+x0,0.75*y0,'S');
      | 
      | dy=100/2-y0-h/2;
      | 
      | if IS_C2
      |     plot([1 1]*(2*x0+w*0.5), 100-y0 - [0 dy]);
      |     plot([1 1]*(2*x0+w*0.5), y0 + [0 dy]);
      |     plot([-1 1]*w/4+(2*x0+w*0.5),(50-h/2)*[1 1])
      |     plot([-1 1]*w/4+(2*x0+w*0.5),(50+h/2)*[1 1])
      | end
      | if IS_C1
      |     plot([1 1]*(2*x0+w*2.5), 100-y0 - [0 dy]);
      |     plot([1 1]*(2*x0+w*2.5), y0 + [0 dy]);
      |     plot([-1 1]*w/4+(2*x0+w*2.5),(50-h/2)*[1 1])
      |     plot([-1 1]*w/4+(2*x0+w*2.5),(50+h/2)*[1 1])
      | end
      | 
      | w=8;
      | x0=102;
      | y0=31;
      | 
      | plot(x0+w*[2 7/3 5/3 2], y0+w*[3.5 2 2 3.5]);
      | 
      | plot(x0+w*[2 2],y0+w*[1 2]);
      | plot(x0+w*[2 2],y0+w*[3.5 4.5]);
      | 
      | plot(x0+w*[1 2],y0+w*[1 1])
      | plot(x0+w*[1 2],y0+w*[4.5 4.5])
      | 
      | plot(x0+w*[1 1],y0+w*[4 5.5])
      | plot(x0+w*[1 1],y0+w*[0 1.5])
      | 
      | plot(x0+w*[1 0.5],y0+w*[4 3])
      | plot(x0+w*[1 0.5],y0+w*[1.5 2.5])
      | plot(x0+w*[0.5 0.5],y0+w*[2 3.5])
      | plot(x0+w*[0.4 0.4],y0+w*[2 3.5])
      | plot(x0+w*[0 0.4],y0+w*[2.75 2.75])
      | 
      | w=8;
      | x0=102;
      | y0=31+w*5.5;
      | 
      | plot(x0+w*[2 7/3 5/3 2], y0+w*[3.5 2 2 3.5]);
      | 
      | plot(x0+w*[2 2],y0+w*[1 2]);
      | plot(x0+w*[2 2],y0+w*[3.5 4.5]);
      | 
      | plot(x0+w*[1 2],y0+w*[1 1])
      | plot(x0+w*[1 2],y0+w*[4.5 4.5])
      | 
      | plot(x0+w*[1 1],y0+w*[4 5.5])
      | plot(x0+w*[1 1],y0+w*[0 1.5])
      | 
      | plot(x0+w*[1 0.5],y0+w*[4 3])
      | plot(x0+w*[1 0.5],y0+w*[1.5 2.5])
      | plot(x0+w*[0.5 0.5],y0+w*[2 3.5])
      | plot(x0+w*[0.4 0.4],y0+w*[2 3.5])
      | plot(x0+w*[0 0.4],y0+w*[2.75 2.75])
      | 
      | port_label('input',1,'ctrl')
      | port_label('output',1,'meas')
      | port_label('rconn',1,'+')
      | port_label('rconn',2,'-')
      | port_label('rconn',3,'S')
      | 
      | port_label('lconn',1,'-')
      | port_label('lconn',2,'N')
  bridgefilter_1ph_PWMblock : Subsystem  mask{LCFilterChoice=LC, L1=L1, R_L1=R_L1, C1=C1, R_C1=R_C1, L2=L2, R_L2=R_L2, C2=C2, R_C2=R_C2, PWM_f=PWM_f, DT=DT, I_MAX=200, I_BACK=183}
      mask prompts: LCFilterChoice "AC-Filter"; L1 "Inductance L1 [H]"; R_L1 "Series resistance of L1 [Ohm]"; C1 "Capacitance C1 [F]"; R_C1 "Series resistance of C1 [Ohm]"; L2 "Inductance L2 [H]"; R_L2 "Series resistance of L2 [Ohm]"; C2 "Capacitance C2 [F]"; R_C2 "Series resistance of C2 [Ohm]"; PWM_f "PWM Frequency"; DT "On Delay"; I_MAX "Blocking Start Current [A]"; I_BACK "Blocking End Current [A]"
      mask init: same as TriphaseHardwaremodule/bridgefilter_1ph
      mask TypeOptions LCFilterChoice: LC | LCL | LCC | LCLC
      mask DialogControl LC Prompt: LC(L)(C)
      mask DialogControl GrpLC Prompt: LC(L)(C)-Filter
      mask DialogControl SW Prompt: Swichted
      mask DialogControl GrpSW Prompt: Switched
      mask Display:
      | IS_L1=true;
      | IS_C1=true;
      | switch get_param(gcb,'LCFilterChoice');
      |     case 'LC'
      |         LCFilterString='LC';
      |         IS_L2=false;
      |         IS_C2=false;
      |     case 'LCL'
      |         LCFilterString='LCL';
      |         IS_L2=true;
      |         IS_C2=false;
      |     case 'LCC'
      |         LCFilterString='LCC';
      |         IS_L2=false;
      |         IS_C2=true;
      |     case 'LCLC'
      |         LCFilterString='LCLC';
      |         IS_L2=true;
      |         IS_C2=true;
      |     otherwise
      |         LCFilterString='LC';
      |         IS_L2=false;
      |         IS_C2=false;
      | end
      | 
      | x0=10;
      | y0=25;
      | w=20;%Breite der Bauelemente
      | h=5;%Höhe der Bauelemente
      | 
      | x1 = linspace(0,1,50);
      | y1 = h*abs(sin(4*pi*x1));
      | 
      | plot(0,0);
      | plot(4*w+4*x0+50,150);
      | 
      | plot(0*w+x0+[0 x0],(100-y0)*[1 1]);
      | plot(0*w+2*x0+[0 w],(100-y0)*[1 1]);
      | if IS_L2
      |     plot(1*w+2*x0+w*x1, y1+100-y0);
      | else
      |     plot(1*w+2*x0+[0 w],(100-y0)*[1 1]);
      | end
      | plot(2*w+2*x0+[0 w],(100-y0)*[1 1]);
      | if IS_L1
      |     plot(3*w+2*x0+w*x1,y1+100-y0);
      | else
      |     plot(3*w+2*x0+[0 w],(100-y0)*[1 1]);
      | end
      | plot(4*w+2*x0+[0 x0],(100-y0)*[1 1]);
      | plot(x0+[0 x0],(y0)*[1 1]);
      | plot(w+x0+[0 7*w],(y0)*[1 1]);
      | 
      | %text(2*w+x0,0.75*y0,'S');
      | 
      | dy=100/2-y0-h/2;
      | 
      | if IS_C2
      |     plot([1 1]*(2*x0+w*0.5), 100-y0 - [0 dy]);
      |     plot([1 1]*(2*x0+w*0.5), y0 + [0 dy]);
      |     plot([-1 1]*w/4+(2*x0+w*0.5),(50-h/2)*[1 1])
      |     plot([-1 1]*w/4+(2*x0+w*0.5),(50+h/2)*[1 1])
      | end
      | if IS_C1
      |     plot([1 1]*(2*x0+w*2.5), 100-y0 - [0 dy]);
      |     plot([1 1]*(2*x0+w*2.5), y0 + [0 dy]);
      |     plot([-1 1]*w/4+(2*x0+w*2.5),(50-h/2)*[1 1])
      |     plot([-1 1]*w/4+(2*x0+w*2.5),(50+h/2)*[1 1])
      | end
      | 
      | w=8;
      | x0=102;
      | y0=31;
      | 
      | plot(x0+w*[2 7/3 5/3 2], y0+w*[3.5 2 2 3.5]);
      | 
      | plot(x0+w*[2 2],y0+w*[1 2]);
      | plot(x0+w*[2 2],y0+w*[3.5 4.5]);
      | 
      | plot(x0+w*[1 2],y0+w*[1 1])
      | plot(x0+w*[1 2],y0+w*[4.5 4.5])
      | 
      | plot(x0+w*[1 1],y0+w*[4 5.5])
      | plot(x0+w*[1 1],y0+w*[0 1.5])
      | 
      | plot(x0+w*[1 0.5],y0+w*[4 3])
      | plot(x0+w*[1 0.5],y0+w*[1.5 2.5])
      | plot(x0+w*[0.5 0.5],y0+w*[2 3.5])
      | plot(x0+w*[0.4 0.4],y0+w*[2 3.5])
      | plot(x0+w*[0 0.4],y0+w*[2.75 2.75])
      | 
      | w=8;
      | x0=102;
      | y0=31+w*5.5;
      | 
      | plot(x0+w*[2 7/3 5/3 2], y0+w*[3.5 2 2 3.5]);
      | 
      | plot(x0+w*[2 2],y0+w*[1 2]);
      | plot(x0+w*[2 2],y0+w*[3.5 4.5]);
      | 
      | plot(x0+w*[1 2],y0+w*[1 1])
      | plot(x0+w*[1 2],y0+w*[4.5 4.5])
      | 
      | plot(x0+w*[1 1],y0+w*[4 5.5])
      | plot(x0+w*[1 1],y0+w*[0 1.5])
      | 
      | plot(x0+w*[1 0.5],y0+w*[4 3])
      | plot(x0+w*[1 0.5],y0+w*[1.5 2.5])
      | plot(x0+w*[0.5 0.5],y0+w*[2 3.5])
      | plot(x0+w*[0.4 0.4],y0+w*[2 3.5])
      | plot(x0+w*[0 0.4],y0+w*[2.75 2.75])
      | 
      | port_label('input',1,'ctrl')
      | port_label('output',1,'meas')
      | port_label('rconn',1,'+')
      | port_label('rconn',2,'-')
      | port_label('rconn',3,'S')
      | 
      | port_label('lconn',1,'-')
      | port_label('lconn',2,'N')
  ctrlSelect2 : Subsystem
  ctrlSelect3 : Subsystem
  ctrlSelect4 : Subsystem
  emptyCtrl : Subsystem
  emptyMeasure : Subsystem
  measMerge2 : Subsystem
  measMerge3 : Subsystem
  measMerge4 : Subsystem
  wires:
  emptyCtrl/1(ctrl) -> ctrlSelect3/1(ctrl), ctrlSelect4/1(ctrl), ctrlSelect2/1(ctrl)
  emptyMeasure/1(meas) -> measMerge4/4(meas4), measMerge4/3(meas3), measMerge4/2(meas2), measMerge4/1(meas1), measMerge3/3(meas3), measMerge3/2(meas2), measMerge3/1(meas1), measMerge2/2(meas2), measMerge2/1(meas1)

== system TriphaseHardwaremodule/ADC-Emulator_F ==
  meas : Inport
  Bus Creator : BusCreator  Inputs=8
  Bus Selector : BusSelector  OutputSignals=meas_u_dc,meas_u_inverter,meas_u_cap,meas_u_out,meas_i_inverter,meas_i_out,connection_state,enabled
  Rate Transition : RateTransition  Integrity=off  InitialCondition=-1  OutPortSampleTime=ControlSampleTime
  Rate Transition1 : RateTransition  Integrity=off  InitialCondition=-1  OutPortSampleTime=ControlSampleTime
  adc_i_inverter : $bdroot/adc  ADC_Emulation=off  ControlSampleTime=ControlSampleTime  HWSampleTime=HWSampleTime  MeasMax=Iac_max  MeasBits=Iac_bit
  adc_i_out : $bdroot/adc  ADC_Emulation=off  ControlSampleTime=ControlSampleTime  HWSampleTime=HWSampleTime  MeasMax=Iac_max  MeasBits=Iac_bit
  adc_u_cap : $bdroot/adc  ADC_Emulation=off  ControlSampleTime=ControlSampleTime  HWSampleTime=HWSampleTime  MeasMax=Vac_max  MeasBits=Vac_bit
  adc_u_dc : $bdroot/adc  ADC_Emulation=off  ControlSampleTime=ControlSampleTime  HWSampleTime=HWSampleTime  MeasMax=Vdc_max  MeasBits=Vdc_bit
  adc_u_inverter : $bdroot/adc  ADC_Emulation=off  ControlSampleTime=ControlSampleTime  HWSampleTime=HWSampleTime  MeasMax=Vac_max  MeasBits=Vac_bit
  adc_u_out : $bdroot/adc  ADC_Emulation=off  ControlSampleTime=ControlSampleTime  HWSampleTime=HWSampleTime  MeasMax=Vac_max  MeasBits=Vac_bit
  measOut : Outport  VectorParamsAs1DForOutWhenUnconnected=off
  wires:
  adc_u_inverter/1 -> Bus Creator/2  "meas_u_inverter"
  Bus Selector/2 -> adc_u_inverter/1  "<meas_u_inverter>"
  Bus Selector/3 -> adc_u_cap/1  "<meas_u_cap>"
  Bus Selector/4 -> adc_u_out/1  "<meas_u_out>"
  Bus Selector/6 -> adc_i_out/1  "<meas_i_out>"
  Bus Selector/5 -> adc_i_inverter/1  "<meas_i_inverter>"
  meas/1 -> Bus Selector/1
  Bus Selector/7 -> Rate Transition/1  "<connection_state>"
  Bus Selector/8 -> Rate Transition1/1  "<enabled>"
  adc_u_dc/1 -> Bus Creator/1  "meas_u_dc"
  adc_i_inverter/1 -> Bus Creator/5  "meas_i_inverter"
  adc_i_out/1 -> Bus Creator/6  "meas_i_out"
  adc_u_out/1 -> Bus Creator/4  "meas_u_out"
  Bus Creator/1 -> measOut/1
  adc_u_cap/1 -> Bus Creator/3  "meas_u_cap"
  Rate Transition/1 -> Bus Creator/7  "connection_state"
  Rate Transition1/1 -> Bus Creator/8  "enabled"
  Bus Selector/1 -> adc_u_dc/1  "<meas_u_dc>"

== system TriphaseHardwaremodule/ADC-Emulator_M ==
  meas : Inport
  Bus Creator : BusCreator  Inputs=2
  Bus Selector : BusSelector  OutputSignals=meas_i_inverter,meas_u_dc
  adc_i_inverter : $bdroot/adc  ADC_Emulation=off  ControlSampleTime=ControlSampleTime  HWSampleTime=HWSampleTime  MeasMax=Iac_max  MeasBits=Iac_bit
  adc_u_dc : $bdroot/adc  ADC_Emulation=off  ControlSampleTime=ControlSampleTime  HWSampleTime=HWSampleTime  MeasMax=Vdc_max  MeasBits=Vdc_bit
  measOut : Outport  VectorParamsAs1DForOutWhenUnconnected=off
  wires:
  Bus Creator/1 -> measOut/1
  adc_u_dc/1 -> Bus Creator/2  "meas_u_dc"
  adc_i_inverter/1 -> Bus Creator/1  "meas_i_inverter"
  meas/1 -> Bus Selector/1
  Bus Selector/1 -> adc_i_inverter/1  "<meas_i_inverter>"
  Bus Selector/2 -> adc_u_dc/1  "<meas_u_dc>"

== system TriphaseHardwaremodule/CommonMode-Filter ==
  Series RLC Branch : powerlib/Elements/Series RLC Branch  LConnTagsString=__new0  RConnTagsString=__new0  BranchType=RLC  Resistance=R_damp  Inductance=L_CM  SetiL0=off  InitialCurrent=0  Capacitance=C_damp  Setx0=off  InitialVoltage=0  Measurements=None
      settings: SourceProductName=Simscape Electrical
  Series RLC Branch1 : powerlib/Elements/Series RLC Branch  LConnTagsString=__new0  RConnTagsString=__new0  BranchType=C  Resistance=1  Inductance=1e-3  SetiL0=off  InitialCurrent=0  Capacitance=C_CM  Setx0=off  InitialVoltage=0  Measurements=None
      settings: SourceProductName=Simscape Electrical
  N : PMIOPort  Side=Left
  M : PMIOPort  Port=2  Side=Right
  connections:
  Series RLC Branch/RConn1 -- M/RConn1 -- Series RLC Branch1/RConn1
  Series RLC Branch/LConn1 -- N/RConn1 -- Series RLC Branch1/LConn1

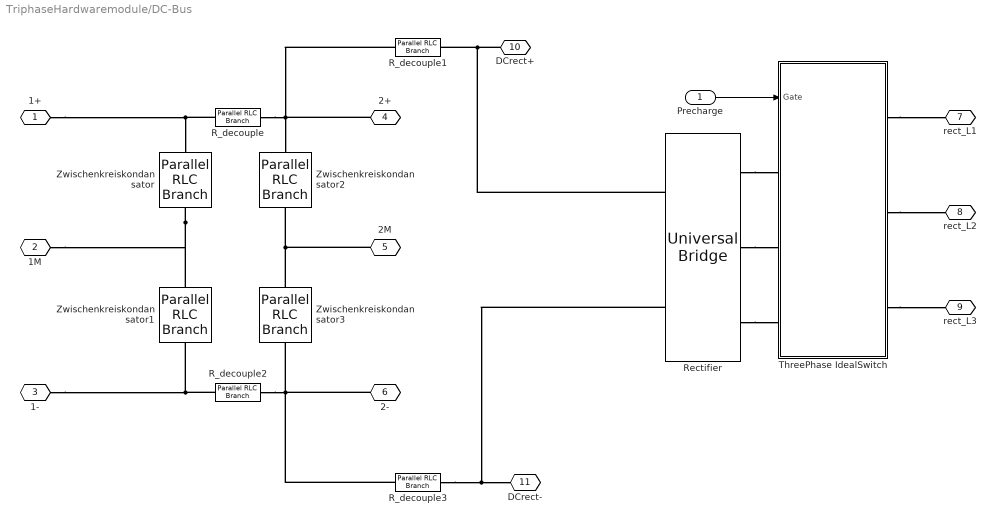
== system TriphaseHardwaremodule/DC-Bus ==
  Precharge : Inport
  R_decouple{,1..3} (4 alike) : powerlib/Elements/Parallel RLC Branch  LConnTagsString=a  RConnTagsString=__new0  BranchType=R  Resistance=1e-3  Inductance=1e-3  SetiL0=off  InitialCurrent=0  Capacitance=C_DC  Setx0=off  InitialVoltage=0  Measurements=None
      settings: SourceProductName=Simscape Electrical
  Rectifier : powerlib/Power Electronics/Universal Bridge  Arms=3  SnubberResistance=1e5  SnubberCapacitance=inf  Device=Diodes  Ron=1e-3  Lon=0  ForwardVoltages="[  0  0  ]"  ForwardVoltage=0  GTOparameters=[ 10e-6 , 20e-6 ]  IGBTparameters=[ 1e-6 , 2e-6 ]  Measurements=None  Measurements_2=None  converterType=Rectifier
      settings: SourceProductName=Simscape Electrical
  ThreePhase IdealSwitch : Subsystem
      mask Display:
      | plot([0 100 100 0 0],[0 0 100 100 0])
      | plot([10 30 60],[30 30 40])
      | plot([10 30 60],[50 50 60])
      | plot([10 30 60],[70 70 80])
      | plot([60 90],[30 30])
      | plot([60 90],[50 50])
      | plot([60 90],[70 70])
  Zwischenkreiskondansator{,1..3} (4 alike) : powerlib/Elements/Parallel RLC Branch  LConnTagsString=a  RConnTagsString=__new0  BranchType=RC  Resistance=R_cap  Inductance=1e-3  SetiL0=off  InitialCurrent=0  Capacitance=C_cap  Setx0=on  InitialVoltage=0  Measurements=None
      settings: SourceProductName=Simscape Electrical
  1+ : PMIOPort  Side=Left
  1M : PMIOPort  Port=2  Side=Left
  1- : PMIOPort  Port=3  Side=Left
  2+ : PMIOPort  Port=4  Side=Left
  2M : PMIOPort  Port=5  Side=Left
  2- : PMIOPort  Port=6  Side=Left
  rect_L1 : PMIOPort  Port=7  Side=Right
  rect_L2 : PMIOPort  Port=8  Side=Right
  rect_L3 : PMIOPort  Port=9  Side=Right
  DCrect+ : PMIOPort  Port=10  Side=Right
  DCrect- : PMIOPort  Port=11  Side=Right
  wires:
  Precharge/1 -> ThreePhase IdealSwitch/1(Gate)
  connections:
  R_decouple3/RConn1 -- Zwischenkreiskondansator3/RConn1 -- 2-/RConn1 -- R_decouple2/LConn1
  R_decouple1/RConn1 -- 2+/RConn1 -- R_decouple/LConn1 -- Zwischenkreiskondansator2/LConn1
  2M/RConn1 -- Zwischenkreiskondansator2/RConn1 -- Zwischenkreiskondansator3/LConn1
  ThreePhase IdealSwitch/RConn1 -- rect_L1/RConn1
  ThreePhase IdealSwitch/RConn2 -- rect_L2/RConn1
  ThreePhase IdealSwitch/RConn3 -- rect_L3/RConn1
  Rectifier/LConn3 -- ThreePhase IdealSwitch/LConn3
  Rectifier/LConn2 -- ThreePhase IdealSwitch/LConn2
  Rectifier/LConn1 -- ThreePhase IdealSwitch/LConn1
  Rectifier/RConn2 -- DCrect-/RConn1 -- R_decouple3/LConn1
  Rectifier/RConn1 -- DCrect+/RConn1 -- R_decouple1/LConn1
  R_decouple2/RConn1 -- 1-/RConn1 -- Zwischenkreiskondansator1/RConn1
  R_decouple/RConn1 -- 1+/RConn1 -- Zwischenkreiskondansator/LConn1
  Zwischenkreiskondansator/RConn1 -- 1M/RConn1 -- Zwischenkreiskondansator1/LConn1

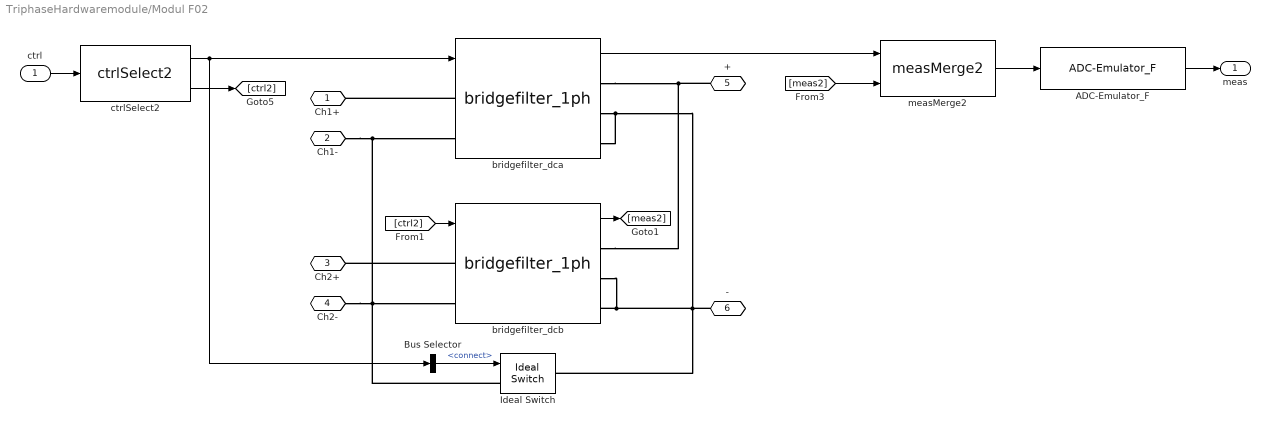
== system TriphaseHardwaremodule/Modul F02 ==
  ctrl : Inport
  ADC-Emulator_F : $bdroot/ADC-Emulator_F  ADC_Emulation=off  ControlSampleTime=ControlSampleTime  HWSampleTime=HWSampleTime  Vac_max=Vac_max  Vac_bit=Vac_bit  Iac_max=Iac_max  Iac_bit=Iac_bit  Vdc_max=Vdc_max  Vdc_bit=Vdc_bit
  Bus Selector : BusSelector  OutputSignals=connect
  Ideal Switch : powerlib/Power Electronics/Ideal Switch  Ron=0.001  Lon=0  IC=0  Rs=1e6  Cs=inf  Measurements=off
      settings: SourceProductName=Simscape Electrical
  bridgefilter_dca : $bdroot/bridgefilter_1ph  LCFilterChoice=LC  L1=L1  R_L1=R_L1  C1=C1  R_C1=R_C1  L2=L2  R_L2=R_L2  C2=C2  R_C2=R_C2  PWM_f=PWM_f  DT=DT
  bridgefilter_dcb : $bdroot/bridgefilter_1ph  LCFilterChoice=LC  L1=L1  R_L1=R_L1  C1=C1  R_C1=R_C1  L2=L2  R_L2=R_L2  C2=C2  R_C2=R_C2  PWM_f=PWM_f  DT=DT
  ctrlSelect2 : $bdroot/ctrlSelect2
  measMerge2 : $bdroot/measMerge2
  Ch1+ : PMIOPort  Tag=PMCPort  Side=Left
  Ch1- : PMIOPort  Tag=PMCPort  Port=2  Side=Left
  Ch2+ : PMIOPort  Tag=PMCPort  Port=3  Side=Left
  Ch2- : PMIOPort  Tag=PMCPort  Port=4  Side=Left
  + : PMIOPort  Tag=PMCPort  Port=5  Side=Right
  - : PMIOPort  Tag=PMCPort  Port=6  Side=Right
  meas : Outport  VectorParamsAs1DForOutWhenUnconnected=off
  wires:
  [ctrl2] -> bridgefilter_dcb/1
  ctrlSelect2/2 -> [ctrl2]
  ctrl/1 -> ctrlSelect2/1
  [meas2] -> measMerge2/2
  bridgefilter_dca/1 -> measMerge2/1
  bridgefilter_dcb/1 -> [meas2]
  ctrlSelect2/1 -> Bus Selector/1, bridgefilter_dca/1
  Bus Selector/1 -> Ideal Switch/1  "<connect>"
  measMerge2/1 -> ADC-Emulator_F/1
  ADC-Emulator_F/1 -> meas/1
  connections:
  bridgefilter_dca/LConn1 -- Ch1+/RConn1
  bridgefilter_dcb/LConn1 -- Ch2+/RConn1
  bridgefilter_dca/RConn1 -- bridgefilter_dcb/RConn1 -- +/RConn1
  bridgefilter_dca/RConn3 -- bridgefilter_dca/RConn2 -- Ideal Switch/RConn1 -- -/RConn1 -- bridgefilter_dcb/RConn2 -- bridgefilter_dcb/RConn3
  Ch2-/RConn1 -- Ideal Switch/LConn1 -- bridgefilter_dca/LConn2 -- Ch1-/RConn1 -- bridgefilter_dcb/LConn2
